simulink model "PWMGenerator"  (R2020b)
settings: Solver=FixedStepAuto  StartTime=0.0  StopTime=0.0001  FixedStep=1e-7  RelTol=1e-3
settings Model: Creator=YiboWang  LastModifiedBy=YiboWang

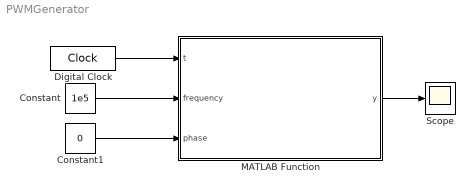
== system PWMGenerator ==
  Constant : Constant  Value=1e5
  Constant1 : Constant  Value=0
  Digital Clock : DigitalClock  SampleTime=1e-7
  MATLAB Function : MATLAB Function  TreatAsAtomicUnit=on  SystemSampleTime=1e-7
  Scope : Scope
  wires:
  Digital Clock/1 -> MATLAB Function/1(t)
  Constant/1 -> MATLAB Function/2(frequency)
  Constant1/1 -> MATLAB Function/3(phase)
  MATLAB Function/1(y) -> Scope/1

== matlab function PWMGenerator/MATLAB Function ==
  data: t input; frequency input; phase input; y output
function y = triangle_wave(t, frequency, phase)
    % 输入: t - 当前仿真时间
    %       frequency - 三角波的频率
    %       phase - 三角波的相位
    % 输出: y - 生成的三角波

    % 计算周期
    T = 1 / frequency;
    
    % 计算相位偏移
    phase_shift = phase * T / (2 * pi);
    
    % 计算三角波
    t_shifted = mod(t + phase_shift, T);
    if t_shifted < T / 2
        y = 4 * t_shifted / T - 1;
    else
        y = 3 - 4 * t_shifted / T;
    end
end
